simulink library "suspensionLib"  (R2022a)
settings: Solver=VariableStepAuto  StartTime=0.0  StopTime=10.0  RelTol=1e-3
undefined symbols (not defined in the file): suspension
settings Model: Creator=grouleau  LastModifiedBy=grouleau

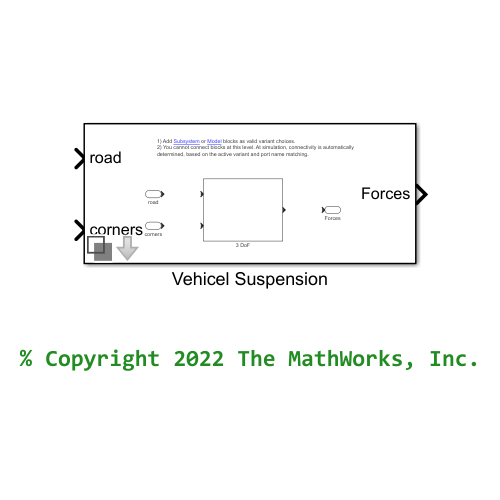
[thumbnail: Simulink's stored preview of the top-level diagram]
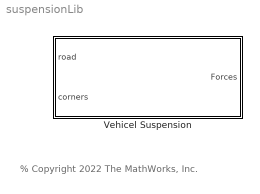
== system suspensionLib ==
  note: % Copyright 2022 The MathWorks, Inc.
  Vehicel Suspension : Subsystem  Variant=on  VariantControlMode=label  LabelModeActiveChoice=suspension.threeDof  mask(slPart){obj=suspension.threeDof}
      mask prompts: obj "slPart Object:"
      mask help: Container block for all slPart blocks
      mask init:
      | obj.maskInit(gcb);

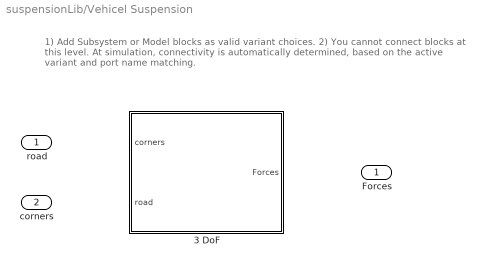
== system suspensionLib/Vehicel Suspension ==
  note: 1) Add Subsystem or Model blocks as valid variant choices.
      | 2) You cannot connect blocks at this level. At simulation, connectivity is automatically
      | determined, based on the active variant and port name matching.
  road : Inport
  corners : Inport  Port=2
  3 DoF : Subsystem  VariantControl=suspension.threeDof
  Forces : Outport

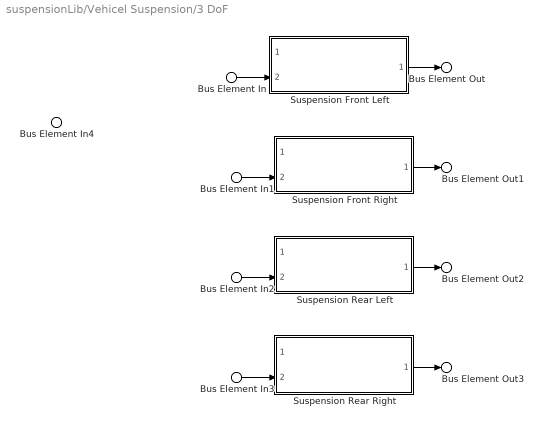
== system suspensionLib/Vehicel Suspension/3 DoF ==
  Bus Element In : Inport  PortName=corners  Element=FrontLeft
  Bus Element In1 : Inport  PortName=corners  Element=FrontRight
  Bus Element In2 : Inport  PortName=corners  Element=RearLeft
  Bus Element In3 : Inport  PortName=corners  Element=RearRight
  Bus Element In4 : Inport  Port=2  PortName=road  Element=signal1
  Suspension Front Left : Subsystem  ReferencedSubsystem=suspension_ss  obj=obj.FrontLeft
      settings: AttributesFormatString=%<obj>
  Suspension Front Right : Subsystem  ReferencedSubsystem=suspension_ss  obj=obj.FrontRight
      settings: AttributesFormatString=%<obj>
  Suspension Rear Left : Subsystem  ReferencedSubsystem=suspension_ss  obj=obj.RearLeft
      settings: AttributesFormatString=%<obj>
  Suspension Rear Right : Subsystem  ReferencedSubsystem=suspension_ss  obj=obj.RearRight
      settings: AttributesFormatString=%<obj>
  Bus Element Out : Outport  PortName=Forces  Element=FrontLeft
  Bus Element Out1 : Outport  PortName=Forces  Element=FrontRight
  Bus Element Out2 : Outport  PortName=Forces  Element=RearLeft
  Bus Element Out3 : Outport  PortName=Forces  Element=RearRight
  wires:
  Bus Element In3/1 -> Suspension Rear Right/2
  Bus Element In2/1 -> Suspension Rear Left/2
  Bus Element In1/1 -> Suspension Front Right/2
  Bus Element In/1 -> Suspension Front Left/2
  Suspension Front Right/1 -> Bus Element Out1/1
  Suspension Front Left/1 -> Bus Element Out/1
  Suspension Rear Right/1 -> Bus Element Out3/1
  Suspension Rear Left/1 -> Bus Element Out2/1
